simulink subsystem "PieroCPModel"  (R2023b)
settings: Solver=VariableStepAuto  StartTime=0.0  StopTime=10.0  RelTol=1e-3
settings Model: Creator=Carlos  LastModifiedBy=Carlos

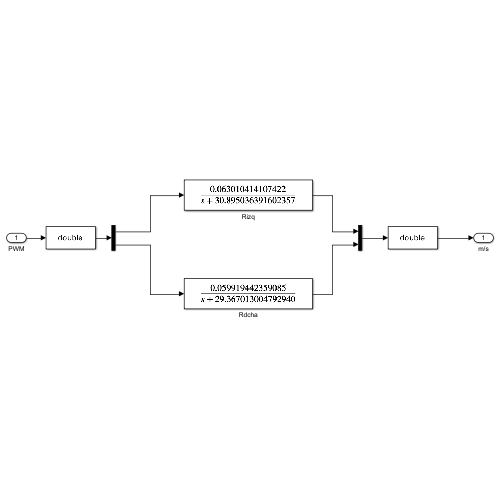
[thumbnail: Simulink's stored preview of the top-level diagram]
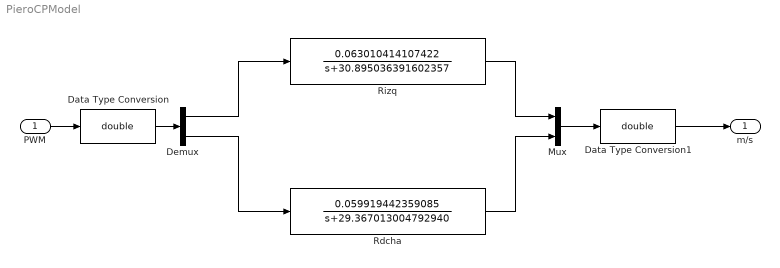
== system PieroCPModel ==
  PWM : Inport
  Data Type Conversion : DataTypeConversion  OutDataTypeStr=double  SaturateOnIntegerOverflow=off  RndMeth=Floor
  Data Type Conversion1 : DataTypeConversion  OutDataTypeStr=double  SaturateOnIntegerOverflow=off  RndMeth=Floor
  Demux : Demux  Outputs=2
  Mux : Mux  Inputs=2
  Rdcha : TransferFcn  Numerator=0.059919442359085  Denominator=[1,29.367013004792940]
  Rizq : TransferFcn  Numerator=0.063010414107422  Denominator=[1,30.895036391602357]
  m/s : Outport
  wires:
  Demux/1 -> Rizq/1
  Demux/2 -> Rdcha/1
  Rizq/1 -> Mux/1
  Rdcha/1 -> Mux/2
  PWM/1 -> Data Type Conversion/1
  Mux/1 -> Data Type Conversion1/1
  Data Type Conversion/1 -> Demux/1
  Data Type Conversion1/1 -> m/s/1
